simulink model "gui1"  (R2016b)
settings: Solver=VariableStepAuto  StartTime=0.0  StopTime=10.0  RelTol=1e-3
undefined symbols (not defined in the file): clientID, jointHandler, mode_blocking, vrep
libraries: simulink x3
settings Model: PauseTimes=1  Creator=crazy  LastModifiedBy=migf1

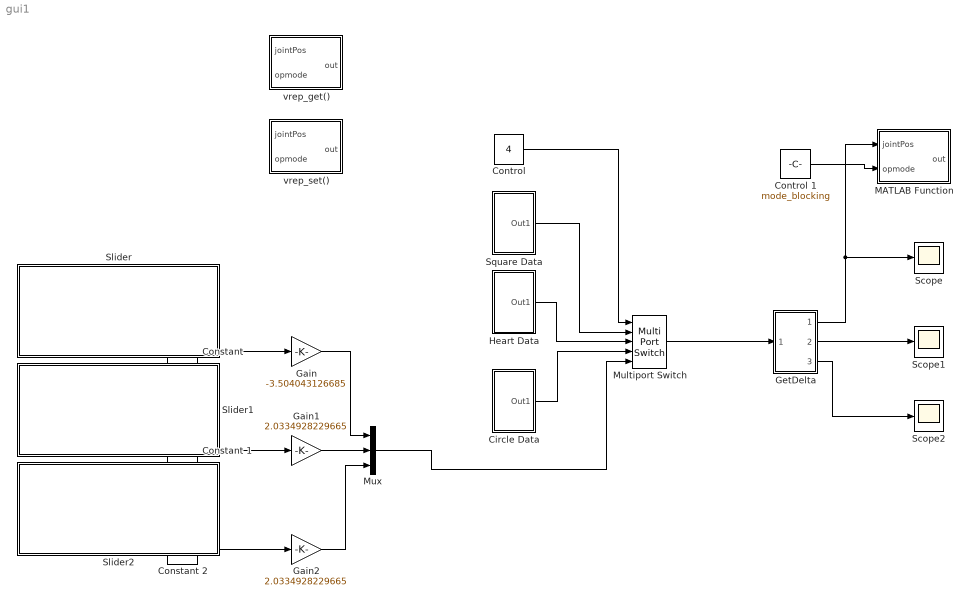
== system gui1 ==
  " GetDelta " : Subsystem
  " Constant " : Constant
  " Constant 1" : Constant
  " Constant 2" : Constant
  "Circle Data " : Subsystem
  "Control " : Constant  Value=4
  Control 1 : Constant  Value=mode_blocking
  Gain : Gain  Gain=-3.504043126685
  Gain1 : Gain  Gain=2.0334928229665
  Gain2 : Gain  Gain=2.0334928229665
  "Heart Data " : Subsystem
  MATLAB Function : MATLAB Function  TreatAsAtomicUnit=on
  Multiport Switch : MultiPortSwitch  Inputs=4
  Mux : Mux  Inputs=3
  Scope : Scope
  Scope1 : Scope
  Scope2 : Scope
  Slider : Subsystem  DialogController=hmiCreateDDGDialog  IsWebBlock=on  mask(MWDashboardBlock){webBlockId=4f94596f-dd6d-4e5e-bddc-7a8d913927f9, webBlockType=slider, ShowInLibBrowser=on, ShowInitialText=on, HMISrcModelName=gui1}
      mask prompts: webBlockId "WebBlock Id"; webBlockType "WebBlock Type"; HMISrcModelName "Source Model"
      mask help: SimulinkHMI:dialogs:SliderDialogDesc
      mask Help: helpview([docroot '/mapfiles/simulink.map'], 'hmi_slider')
      mask Display:
      | if strcmp(get_param(bdroot(gcb),'BlockDiagramType'), 'library')
      |     image([(matlabroot) '/toolbox/simulink/hmi/icons/Slider.png']);
      | end
  Slider1 : Subsystem  DialogController=hmiCreateDDGDialog  IsWebBlock=on  mask(MWDashboardBlock){webBlockId=8aa996ad-7cd4-40fc-9a04-6a85939aea5d, webBlockType=slider, ShowInLibBrowser=on, ShowInitialText=on, HMISrcModelName=gui1}
      mask prompts: webBlockId "WebBlock Id"; webBlockType "WebBlock Type"; HMISrcModelName "Source Model"
      mask help: SimulinkHMI:dialogs:SliderDialogDesc
      mask Help: helpview([docroot '/mapfiles/simulink.map'], 'hmi_slider')
      mask Display:
      | if strcmp(get_param(bdroot(gcb),'BlockDiagramType'), 'library')
      |     image([(matlabroot) '/toolbox/simulink/hmi/icons/Slider.png']);
      | end
  Slider2 : Subsystem  DialogController=hmiCreateDDGDialog  IsWebBlock=on  mask(MWDashboardBlock){webBlockId=1ddf6fd9-0225-4881-82ca-a25e179e2ab9, webBlockType=slider, ShowInLibBrowser=on, ShowInitialText=on, HMISrcModelName=gui1}
      mask prompts: webBlockId "WebBlock Id"; webBlockType "WebBlock Type"; HMISrcModelName "Source Model"
      mask help: SimulinkHMI:dialogs:SliderDialogDesc
      mask Help: helpview([docroot '/mapfiles/simulink.map'], 'hmi_slider')
      mask Display:
      | if strcmp(get_param(bdroot(gcb),'BlockDiagramType'), 'library')
      |     image([(matlabroot) '/toolbox/simulink/hmi/icons/Slider.png']);
      | end
  "Square Data " : Subsystem
  "vrep_get() " : MATLAB Function  TreatAsAtomicUnit=on
  "vrep_set() " : MATLAB Function  TreatAsAtomicUnit=on
  wires:
  " GetDelta "/2(Out2) -> Scope1/1
  " GetDelta "/3(Out3) -> Scope2/1
  Multiport Switch/1 -> " GetDelta "/1(In1)
  "Control "/1 -> Multiport Switch/1
  " Constant "/1 -> Gain/1
  " Constant 1"/1 -> Gain1/1
  " Constant 2"/1 -> Gain2/1
  Gain/1 -> Mux/1
  Gain1/1 -> Mux/2
  Gain2/1 -> Mux/3
  Mux/1 -> Multiport Switch/5
  " GetDelta "/1(Out1) -> Scope/1, MATLAB Function/1(jointPos)
  Control 1/1 -> MATLAB Function/2(opmode)
  "Square Data "/1(Out1) -> Multiport Switch/2
  "Heart Data "/1(Out1) -> Multiport Switch/3
  "Circle Data "/1(Out1) -> Multiport Switch/4

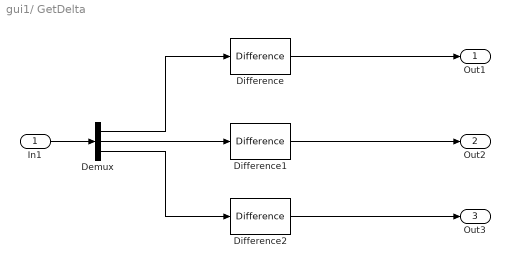
== system gui1/ GetDelta  ==
  In1 : Inport
  Demux : Demux  Outputs=3
  Difference : simulink/Discrete/Difference  ICPrevInput=0  OutMin=[]  OutMax=[]  OutDataType=fixdt(1, 16)  OutScaling=2^-10  DoSatur=off
  Difference1 : simulink/Discrete/Difference  ICPrevInput=0  OutMin=[]  OutMax=[]  OutDataType=fixdt(1, 16)  OutScaling=2^-10  DoSatur=off
  Difference2 : simulink/Discrete/Difference  ICPrevInput=0  OutMin=[]  OutMax=[]  OutDataType=fixdt(1, 16)  OutScaling=2^-10  DoSatur=off
  Out1 : Outport
  Out2 : Outport  Port=2
  Out3 : Outport  Port=3
  wires:
  Difference1/1 -> Out2/1
  Difference/1 -> Out1/1
  Difference2/1 -> Out3/1
  In1/1 -> Demux/1
  Demux/1 -> Difference/1
  Demux/2 -> Difference1/1
  Demux/3 -> Difference2/1

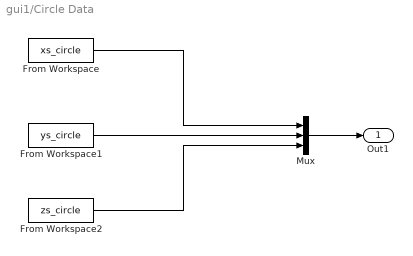
== system gui1/Circle Data  ==
  From Workspace : FromWorkspace  VariableName=xs_circle  SampleTime=1
  From Workspace1 : FromWorkspace  VariableName=ys_circle  SampleTime=1
  From Workspace2 : FromWorkspace  VariableName=zs_circle  SampleTime=1
  Mux : Mux  Inputs=3
  Out1 : Outport
  wires:
  From Workspace/1 -> Mux/1
  From Workspace2/1 -> Mux/3
  Mux/1 -> Out1/1
  From Workspace1/1 -> Mux/2

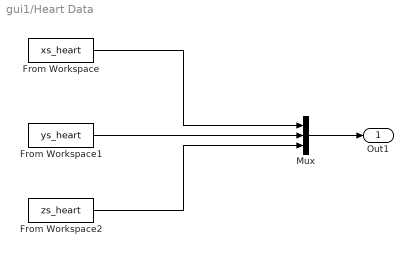
== system gui1/Heart Data  ==
  From Workspace : FromWorkspace  VariableName=xs_heart  SampleTime=1
  From Workspace1 : FromWorkspace  VariableName=ys_heart  SampleTime=1
  From Workspace2 : FromWorkspace  VariableName=zs_heart  SampleTime=1
  Mux : Mux  Inputs=3
  Out1 : Outport
  wires:
  From Workspace/1 -> Mux/1
  From Workspace2/1 -> Mux/3
  Mux/1 -> Out1/1
  From Workspace1/1 -> Mux/2

== system gui1/Slider ==

== system gui1/Slider1 ==

== system gui1/Slider2 ==

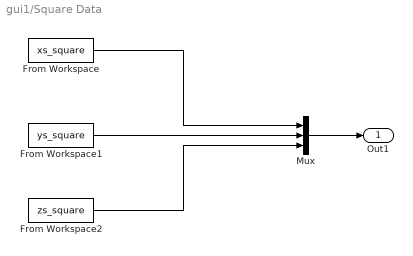
== system gui1/Square Data  ==
  From Workspace : FromWorkspace  VariableName=xs_square  SampleTime=1
  From Workspace1 : FromWorkspace  VariableName=ys_square  SampleTime=1
  From Workspace2 : FromWorkspace  VariableName=zs_square  SampleTime=1
  Mux : Mux  Inputs=3
  Out1 : Outport
  wires:
  From Workspace/1 -> Mux/1
  From Workspace2/1 -> Mux/3
  Mux/1 -> Out1/1
  From Workspace1/1 -> Mux/2

== matlab function gui1/vrep_set()  ==
  data: out output; jointPos input; opmode input; clientID parameter; jointHandler parameter; vrep parameter
function out   = Vrep_setJointPos( jointPos, opmode,  clientID, jointHandler, vrep)
%UNTITLED Summary of this function goes here
%   Detailed explanation goes here
 %global vrep clientID prismaticJointS22;
 % vrep.simx_opmode_blocking
 %vrep object
 %client Id from Vrep
 % joint handler: example prismaticJointS22
 %joinPos[rad]
 %position mode
% global vrep;
 
 [out] = vrep.simxSetJointTargetPosition(clientID, jointHandler, jointPos,opmode);

 

end

== matlab function gui1/MATLAB Function ==
  data: out output; jointPos input; opmode input; clientID parameter; jointHandler parameter; vrep parameter
function out   = Vrep_setJointPos( jointPos, opmode,  clientID, jointHandler, vrep)
%UNTITLED Summary of this function goes here
%   Detailed explanation goes here
 %global vrep clientID prismaticJointS22;
 % vrep.simx_opmode_blocking
 %vrep object
 %client Id from Vrep
 % joint handler: example prismaticJointS22
 %joinPos[rad]
 %position mode
% global vrep;
 
 [out] = vrep.simxSetJointTargetPosition(clientID, jointHandler, jointPos,opmode);

 

end

== matlab function gui1/vrep_get()  ==
  data: out output; jointPos input; opmode input; clientID parameter; jointHandler parameter; vrep parameter
function out   = Vrep_setJointPos( jointPos, opmode,  clientID, jointHandler, vrep)
%UNTITLED Summary of this function goes here
%   Detailed explanation goes here
 %global vrep clientID prismaticJointS22;
 % vrep.simx_opmode_blocking
 %vrep object
 %client Id from Vrep
 % joint handler: example prismaticJointS22
 %joinPos[rad]
 %position mode
% global vrep;
 
 [out] = vrep.simxSetJointTargetPosition(clientID, jointHandler, jointPos,opmode);

 

end
